simulink model "Linear_Decoupled_2nd_Order"  (R2022a)
settings: Solver=VariableStepAuto  StartTime=0  StopTime=1000  RelTol=1e-3
undefined symbols (not defined in the file): A_HD, A_HD2, A_platform, B_HD, B_HD2, B_platform, C_HD, C_HD2, C_platform, HD_op
settings Model: Creator=ianam  LastModifiedBy=ianam
settings DebuggingCC: UnderSpecifiedDataTypeMsg=error  UnderSpecifiedDimensionMsg=error

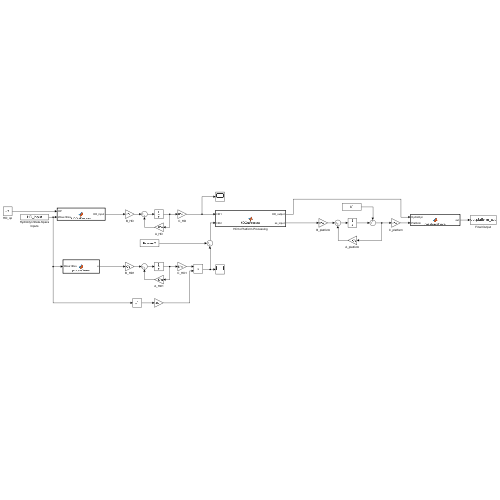
[thumbnail: Simulink's stored preview of the top-level diagram]
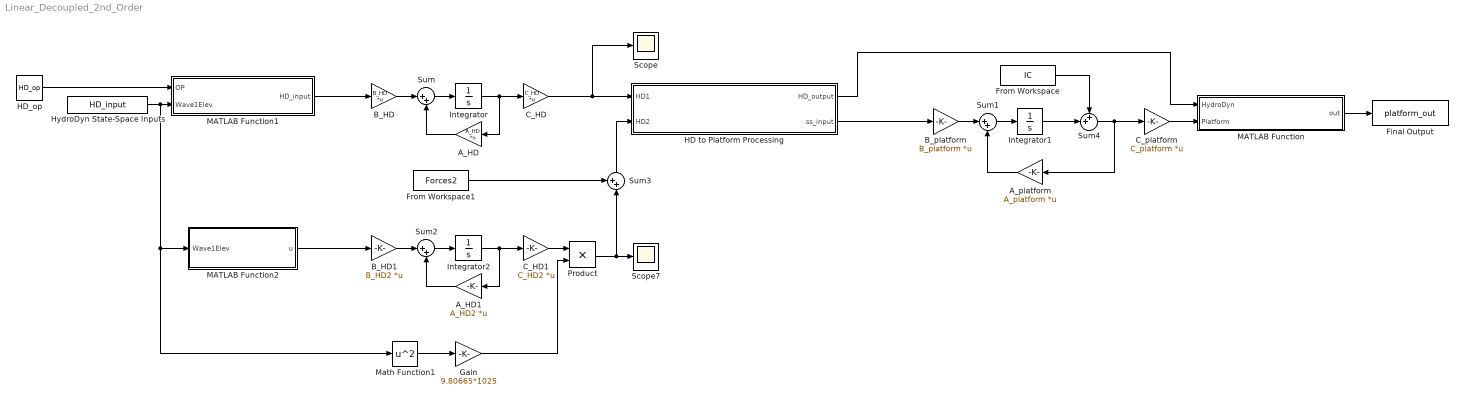
== system Linear_Decoupled_2nd_Order ==
  A_HD : Gain  Gain=A_HD  Multiplication=Matrix(K*u)
  A_HD1 : Gain  Gain=A_HD2  Multiplication=Matrix(K*u)
  A_platform : Gain  Gain=A_platform  Multiplication=Matrix(K*u)
  B_HD : Gain  Gain=B_HD  Multiplication=Matrix(K*u)
  B_HD1 : Gain  Gain=B_HD2  Multiplication=Matrix(K*u)
  B_platform : Gain  Gain=B_platform  Multiplication=Matrix(K*u)
  C_HD : Gain  Gain=C_HD  Multiplication=Matrix(K*u)
  C_HD1 : Gain  Gain=C_HD2  Multiplication=Matrix(K*u)
  C_platform : Gain  Gain=C_platform  Multiplication=Matrix(K*u)
  Final Output : ToWorkspace  VariableName=platform_out  SaveFormat=Timeseries  SampleTime=-1
  From Workspace : FromWorkspace  VariableName=IC
  From Workspace1 : FromWorkspace  VariableName=Forces2
  Gain : Gain  Gain=9.80665*1025
  HD to Platform Processing : MATLAB Function  TreatAsAtomicUnit=on
  HD_op : Constant  Value=HD_op
  HydroDyn State-Space Inputs : FromWorkspace  VariableName=HD_input
  Integrator : Integrator
  Integrator1 : Integrator
  Integrator2 : Integrator
  MATLAB Function : MATLAB Function  TreatAsAtomicUnit=on
  MATLAB Function1 : MATLAB Function  TreatAsAtomicUnit=on
  MATLAB Function2 : MATLAB Function  TreatAsAtomicUnit=on
  Math Function1 : Math  Operator=square
  Product : Product
  Scope : Scope
  Scope7 : Scope
  Sum : Sum  Inputs=|++
  Sum1 : Sum  Inputs=|++
  Sum2 : Sum  Inputs=|++
  Sum3 : Sum  Inputs=++|
  Sum4 : Sum  Inputs=++|
  wires:
  Sum/1 -> Integrator/1
  Integrator/1 -> C_HD/1, A_HD/1
  A_HD/1 -> Sum/2
  B_HD/1 -> Sum/1
  B_platform/1 -> Sum1/1
  Sum1/1 -> Integrator1/1
  A_platform/1 -> Sum1/2
  MATLAB Function1/1(HD_input) -> B_HD/1
  HD_op/1 -> MATLAB Function1/1(OP)
  HD to Platform Processing/2(ss_input) -> B_platform/1
  Sum4/1 -> A_platform/1, C_platform/1
  Integrator1/1 -> Sum4/2
  From Workspace/1 -> Sum4/1
  MATLAB Function/1(out) -> Final Output/1
  C_platform/1 -> MATLAB Function/2(Platform)
  C_HD/1 -> Scope/1, HD to Platform Processing/1(HD1)
  A_HD1/1 -> Sum2/2
  Integrator2/1 -> C_HD1/1, A_HD1/1
  B_HD1/1 -> Sum2/1
  Sum2/1 -> Integrator2/1
  HD to Platform Processing/1(HD_output) -> MATLAB Function/1(HydroDyn)
  MATLAB Function2/1(u) -> B_HD1/1
  C_HD1/1 -> Product/1
  HydroDyn State-Space Inputs/1 -> Math Function1/1, MATLAB Function2/1(Wave1Elev), MATLAB Function1/2(Wave1Elev)
  Math Function1/1 -> Gain/1
  Gain/1 -> Product/2
  Product/1 -> Sum3/2, Scope7/1
  From Workspace1/1 -> Sum3/1
  Sum3/1 -> HD to Platform Processing/2(HD2)

== matlab function Linear_Decoupled_2nd_Order/MATLAB Function1 ==
  data: OP input; Wave1Elev input; HD_input output
function HD_input = HDOutProcess(OP,Wave1Elev)

% Define quantities
% wam_trans = states(1:6);
% wam_vel = states(11:16);

% Create input vector
HD_input = zeros(37,1);

% Assign HD outputs to input vector
% HD_input(1:6) = wam_trans;
% HD_input(7:12) = wam_vel;
HD_input(37) = Wave1Elev;

% Add operating point to inputs
HD_input = HD_input + OP;

end

== matlab function Linear_Decoupled_2nd_Order/HD to Platform Processing ==
  data: HD_output output; HD1 input; ss_input output size=235,1; HD2 input
function [HD_output,ss_input] = HDOutProcess(HD1,HD2)

% Initialize
HydroF = zeros(6,1);
HD_output = zeros(25,1);

% Define quantities
Wave1Elev = HD1(1);
HydroF(1) = HD1(2) + HD2(1);
HydroF(2) = HD1(3) + HD2(2);
HydroF(3) = HD1(4) + HD2(3);
HydroF(4) = HD1(5) + HD2(4);
HydroF(5) = HD1(6) + HD2(5);
HydroF(6) = HD1(7) + HD2(6);

HD_output(:,1) = HD1(:);
HD_output(2:7) = HD_output(2:7) + HD2(1:6);
HD_output(8:13) = HD_output(8:13) + HD2(1:6);
HD_output(20:25) = HD2(1:6);

% Create input vector
ss_input = zeros(235,1);

% Assign HD outputs to input vector
ss_input(40:45,1) = HydroF(:,1);

ss_input(226,1) = Wave1Elev(1);

end

== matlab function Linear_Decoupled_2nd_Order/MATLAB Function ==
  data: HydroDyn input; out output; Platform input
function out = passWaveForce(HydroDyn,Platform)

% Read Forces from HydroDyn Output
force = HydroDyn(2:end,1);

% Add Forces to Total Output
Platform(34:57,1) = force;

out = Platform;

end

== matlab function Linear_Decoupled_2nd_Order/MATLAB Function2 ==
  data: Wave1Elev input; u output
function u = processWave(Wave1Elev)

u = repmat(Wave1Elev,6,1);

end
